simulink library "AtomicLibrary"
PostLoadFcn:
  | PacketBusGenerator; RailCabBusGenerator
(part 4 of 8)

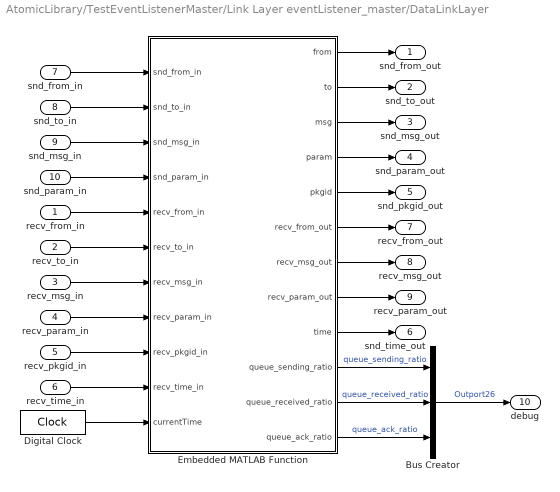
== system AtomicLibrary/TestEventListenerMaster/Link Layer eventListener_master/DataLinkLayer ==
  recv_from_in : Inport  Tag=id=_q-qdMPdmEeGH_6eRdlYQdA  Port=1  PortDimensions=-1  DataType=uint8  OutDataType=fixdt(1, 16)  OutScaling=2^0  OutDataTypeStr=uint8
  recv_to_in : Inport  Tag=id=_q-rrUPdmEeGH_6eRdlYQdA  Port=2  PortDimensions=-1  DataType=uint8  OutDataType=fixdt(1, 16)  OutScaling=2^0  OutDataTypeStr=uint8
  recv_msg_in : Inport  Tag=id=_q-sSYPdmEeGH_6eRdlYQdA  Port=3  PortDimensions=-1  DataType=uint16  OutDataType=fixdt(1, 16)  OutScaling=2^0  OutDataTypeStr=uint16
  recv_param_in : Inport  Tag=id=_q-tggPdmEeGH_6eRdlYQdA  Port=4  PortDimensions=-1  DataType=double  OutDataType=fixdt(1, 16)  OutScaling=2^0  OutDataTypeStr=double
  recv_pkgid_in : Inport  Tag=id=_q-uuoPdmEeGH_6eRdlYQdA  Port=5  PortDimensions=-1  DataType=uint32  OutDataType=fixdt(1, 16)  OutScaling=2^0  OutDataTypeStr=uint32
  recv_time_in : Inport  Tag=id=_q-v8wPdmEeGH_6eRdlYQdA  Port=6  PortDimensions=-1  DataType=double  OutDataType=fixdt(1, 16)  OutScaling=2^0  OutDataTypeStr=double
  snd_from_in : Inport  Tag=id=_q-wj0PdmEeGH_6eRdlYQdA  Port=7  PortDimensions=-1  DataType=uint8  OutDataType=fixdt(1, 16)  OutScaling=2^0  OutDataTypeStr=uint8
  snd_to_in : Inport  Tag=id=_q-xx8PdmEeGH_6eRdlYQdA  Port=8  PortDimensions=-1  DataType=uint8  OutDataType=fixdt(1, 16)  OutScaling=2^0  OutDataTypeStr=uint8
  snd_msg_in : Inport  Tag=id=_q-zAEPdmEeGH_6eRdlYQdA  Port=9  PortDimensions=-1  DataType=uint16  OutDataType=fixdt(1, 16)  OutScaling=2^0  OutDataTypeStr=uint16
  snd_param_in : Inport  Tag=id=_q-01QPdmEeGH_6eRdlYQdA  Port=10  PortDimensions=-1  DataType=double  OutDataType=fixdt(1, 16)  OutScaling=2^0  OutDataTypeStr=double
  snd_from_out : Outport  Tag=id=_q-gFIPdmEeGH_6eRdlYQdA  Port=1  PortDimensions=-1  DataType=uint8  OutDataType=fixdt(1, 16)  OutScaling=2^0  OutDataTypeStr=uint8
  snd_to_out : Outport  Tag=id=_q-gsMPdmEeGH_6eRdlYQdA  Port=2  PortDimensions=-1  DataType=uint8  OutDataType=fixdt(1, 16)  OutScaling=2^0  OutDataTypeStr=uint8
  snd_msg_out : Outport  Tag=id=_q-hTQPdmEeGH_6eRdlYQdA  Port=3  PortDimensions=-1  DataType=uint16  OutDataType=fixdt(1, 16)  OutScaling=2^0  OutDataTypeStr=uint16
  snd_param_out : Outport  Tag=id=_q-ihYPdmEeGH_6eRdlYQdA  Port=4  PortDimensions=-1  DataType=double  OutDataType=fixdt(1, 16)  OutScaling=2^0  OutDataTypeStr=double
  snd_pkgid_out : Outport  Tag=id=_q-jvgPdmEeGH_6eRdlYQdA  Port=5  PortDimensions=-1  DataType=uint32  OutDataType=fixdt(1, 16)  OutScaling=2^0  OutDataTypeStr=uint32
  snd_time_out : Outport  Tag=id=_q-k9oPdmEeGH_6eRdlYQdA  Port=6  PortDimensions=-1  DataType=double  OutDataType=fixdt(1, 16)  OutScaling=2^0  OutDataTypeStr=double
  recv_from_out : Outport  Tag=id=_q-mLwPdmEeGH_6eRdlYQdA  Port=7  PortDimensions=-1  DataType=uint8  OutDataType=fixdt(1, 16)  OutScaling=2^0  OutDataTypeStr=uint8
  recv_msg_out : Outport  Tag=id=_q-nZ4PdmEeGH_6eRdlYQdA  Port=8  PortDimensions=-1  DataType=uint16  OutDataType=fixdt(1, 16)  OutScaling=2^0  OutDataTypeStr=uint16
  recv_param_out : Outport  Tag=id=_q-oA8PdmEeGH_6eRdlYQdA  Port=9  PortDimensions=-1  DataType=double  OutDataType=fixdt(1, 16)  OutScaling=2^0  OutDataTypeStr=double
  debug : Outport  Tag=id=_q-pPEPdmEeGH_6eRdlYQdA  Port=10  PortDimensions=-1  DataType=auto  OutDataType=fixdt(1, 16)  OutScaling=2^0  OutDataTypeStr=Inherit: auto
  Bus Creator : BusCreator  Inputs=3  Tag=id=_q-2DYPdmEeGH_6eRdlYQdA
  Embedded MATLAB Function : Stateflow chart  Tag=id=_q-2DYfdmEeGH_6eRdlYQdA
  Digital Clock : DigitalClock  Tag=id=_q-5GsPdmEeGH_6eRdlYQdA  SampleTime=0.1
  wires:
  Embedded MATLAB Function/12(queue_ack_ratio) -> Bus Creator/3  "queue_ack_ratio"
  Embedded MATLAB Function/10(queue_sending_ratio) -> Bus Creator/1  "queue_sending_ratio"
  Embedded MATLAB Function/8(recv_param_out) -> recv_param_out/1
  recv_to_in/1 -> Embedded MATLAB Function/6(recv_to_in)
  Embedded MATLAB Function/5(pkgid) -> snd_pkgid_out/1
  snd_from_in/1 -> Embedded MATLAB Function/1(snd_from_in)
  Embedded MATLAB Function/7(recv_msg_out) -> recv_msg_out/1
  recv_pkgid_in/1 -> Embedded MATLAB Function/9(recv_pkgid_in)
  snd_msg_in/1 -> Embedded MATLAB Function/3(snd_msg_in)
  Digital Clock/1 -> Embedded MATLAB Function/11(currentTime)
  Embedded MATLAB Function/3(msg) -> snd_msg_out/1
  Embedded MATLAB Function/9(time) -> snd_time_out/1
  recv_from_in/1 -> Embedded MATLAB Function/5(recv_from_in)
  recv_time_in/1 -> Embedded MATLAB Function/10(recv_time_in)
  snd_to_in/1 -> Embedded MATLAB Function/2(snd_to_in)
  snd_param_in/1 -> Embedded MATLAB Function/4(snd_param_in)
  Embedded MATLAB Function/6(recv_from_out) -> recv_from_out/1
  recv_param_in/1 -> Embedded MATLAB Function/8(recv_param_in)
  Embedded MATLAB Function/2(to) -> snd_to_out/1
  recv_msg_in/1 -> Embedded MATLAB Function/7(recv_msg_in)
  Embedded MATLAB Function/4(param) -> snd_param_out/1
  Embedded MATLAB Function/1(from) -> snd_from_out/1
  Bus Creator/1 -> debug/1  "Outport26"
  Embedded MATLAB Function/11(queue_received_ratio) -> Bus Creator/2  "queue_received_ratio"

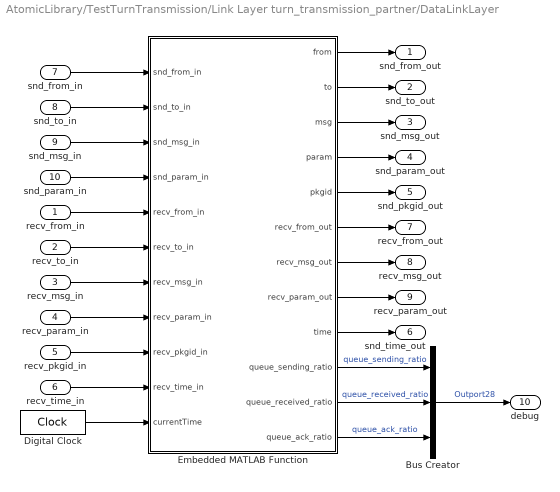
== system AtomicLibrary/TestTurnTransmission/Link Layer turn_transmission_partner/DataLinkLayer ==
  recv_from_in : Inport  Tag=id=_rHclwPdmEeGH_6eRdlYQdA  Port=1  PortDimensions=-1  DataType=uint8  OutDataType=fixdt(1, 16)  OutScaling=2^0  OutDataTypeStr=uint8
  recv_to_in : Inport  Tag=id=_rHdz4PdmEeGH_6eRdlYQdA  Port=2  PortDimensions=-1  DataType=uint8  OutDataType=fixdt(1, 16)  OutScaling=2^0  OutDataTypeStr=uint8
  recv_msg_in : Inport  Tag=id=_rHfCAPdmEeGH_6eRdlYQdA  Port=3  PortDimensions=-1  DataType=uint16  OutDataType=fixdt(1, 16)  OutScaling=2^0  OutDataTypeStr=uint16
  recv_param_in : Inport  Tag=id=_rHfpEPdmEeGH_6eRdlYQdA  Port=4  PortDimensions=-1  DataType=double  OutDataType=fixdt(1, 16)  OutScaling=2^0  OutDataTypeStr=double
  recv_pkgid_in : Inport  Tag=id=_rHg3MPdmEeGH_6eRdlYQdA  Port=5  PortDimensions=-1  DataType=uint32  OutDataType=fixdt(1, 16)  OutScaling=2^0  OutDataTypeStr=uint32
  recv_time_in : Inport  Tag=id=_rHiFUPdmEeGH_6eRdlYQdA  Port=6  PortDimensions=-1  DataType=double  OutDataType=fixdt(1, 16)  OutScaling=2^0  OutDataTypeStr=double
  snd_from_in : Inport  Tag=id=_rHjTcPdmEeGH_6eRdlYQdA  Port=7  PortDimensions=-1  DataType=uint8  OutDataType=fixdt(1, 16)  OutScaling=2^0  OutDataTypeStr=uint8
  snd_to_in : Inport  Tag=id=_rHkhkPdmEeGH_6eRdlYQdA  Port=8  PortDimensions=-1  DataType=uint8  OutDataType=fixdt(1, 16)  OutScaling=2^0  OutDataTypeStr=uint8
  snd_msg_in : Inport  Tag=id=_rHlIoPdmEeGH_6eRdlYQdA  Port=9  PortDimensions=-1  DataType=uint16  OutDataType=fixdt(1, 16)  OutScaling=2^0  OutDataTypeStr=uint16
  snd_param_in : Inport  Tag=id=_rHmWwPdmEeGH_6eRdlYQdA  Port=10  PortDimensions=-1  DataType=double  OutDataType=fixdt(1, 16)  OutScaling=2^0  OutDataTypeStr=double
  snd_from_out : Outport  Tag=id=_rHRmoPdmEeGH_6eRdlYQdA  Port=1  PortDimensions=-1  DataType=uint8  OutDataType=fixdt(1, 16)  OutScaling=2^0  OutDataTypeStr=uint8
  snd_to_out : Outport  Tag=id=_rHS0wPdmEeGH_6eRdlYQdA  Port=2  PortDimensions=-1  DataType=uint8  OutDataType=fixdt(1, 16)  OutScaling=2^0  OutDataTypeStr=uint8
  snd_msg_out : Outport  Tag=id=_rHTb0PdmEeGH_6eRdlYQdA  Port=3  PortDimensions=-1  DataType=uint16  OutDataType=fixdt(1, 16)  OutScaling=2^0  OutDataTypeStr=uint16
  snd_param_out : Outport  Tag=id=_rHUp8PdmEeGH_6eRdlYQdA  Port=4  PortDimensions=-1  DataType=double  OutDataType=fixdt(1, 16)  OutScaling=2^0  OutDataTypeStr=double
  snd_pkgid_out : Outport  Tag=id=_rHVRAPdmEeGH_6eRdlYQdA  Port=5  PortDimensions=-1  DataType=uint32  OutDataType=fixdt(1, 16)  OutScaling=2^0  OutDataTypeStr=uint32
  snd_time_out : Outport  Tag=id=_rHWfIPdmEeGH_6eRdlYQdA  Port=6  PortDimensions=-1  DataType=double  OutDataType=fixdt(1, 16)  OutScaling=2^0  OutDataTypeStr=double
  recv_from_out : Outport  Tag=id=_rHXGMPdmEeGH_6eRdlYQdA  Port=7  PortDimensions=-1  DataType=uint8  OutDataType=fixdt(1, 16)  OutScaling=2^0  OutDataTypeStr=uint8
  recv_msg_out : Outport  Tag=id=_rHYUUPdmEeGH_6eRdlYQdA  Port=8  PortDimensions=-1  DataType=uint16  OutDataType=fixdt(1, 16)  OutScaling=2^0  OutDataTypeStr=uint16
  recv_param_out : Outport  Tag=id=_rHZicPdmEeGH_6eRdlYQdA  Port=9  PortDimensions=-1  DataType=double  OutDataType=fixdt(1, 16)  OutScaling=2^0  OutDataTypeStr=double
  debug : Outport  Tag=id=_rHawkPdmEeGH_6eRdlYQdA  Port=10  PortDimensions=-1  DataType=auto  OutDataType=fixdt(1, 16)  OutScaling=2^0  OutDataTypeStr=Inherit: auto
  Bus Creator : BusCreator  Inputs=3  Tag=id=_rHoL8PdmEeGH_6eRdlYQdA
  Embedded MATLAB Function : Stateflow chart  Tag=id=_rHoL8fdmEeGH_6eRdlYQdA
  Digital Clock : DigitalClock  Tag=id=_rHqoMPdmEeGH_6eRdlYQdA  SampleTime=0.1
  wires:
  Embedded MATLAB Function/12(queue_ack_ratio) -> Bus Creator/3  "queue_ack_ratio"
  Embedded MATLAB Function/10(queue_sending_ratio) -> Bus Creator/1  "queue_sending_ratio"
  Embedded MATLAB Function/8(recv_param_out) -> recv_param_out/1
  recv_to_in/1 -> Embedded MATLAB Function/6(recv_to_in)
  Embedded MATLAB Function/5(pkgid) -> snd_pkgid_out/1
  snd_from_in/1 -> Embedded MATLAB Function/1(snd_from_in)
  Embedded MATLAB Function/7(recv_msg_out) -> recv_msg_out/1
  recv_pkgid_in/1 -> Embedded MATLAB Function/9(recv_pkgid_in)
  snd_msg_in/1 -> Embedded MATLAB Function/3(snd_msg_in)
  Digital Clock/1 -> Embedded MATLAB Function/11(currentTime)
  Embedded MATLAB Function/3(msg) -> snd_msg_out/1
  Embedded MATLAB Function/9(time) -> snd_time_out/1
  recv_from_in/1 -> Embedded MATLAB Function/5(recv_from_in)
  recv_time_in/1 -> Embedded MATLAB Function/10(recv_time_in)
  snd_to_in/1 -> Embedded MATLAB Function/2(snd_to_in)
  snd_param_in/1 -> Embedded MATLAB Function/4(snd_param_in)
  Embedded MATLAB Function/6(recv_from_out) -> recv_from_out/1
  recv_param_in/1 -> Embedded MATLAB Function/8(recv_param_in)
  Embedded MATLAB Function/2(to) -> snd_to_out/1
  recv_msg_in/1 -> Embedded MATLAB Function/7(recv_msg_in)
  Embedded MATLAB Function/4(param) -> snd_param_out/1
  Embedded MATLAB Function/1(from) -> snd_from_out/1
  Bus Creator/1 -> debug/1  "Outport28"
  Embedded MATLAB Function/11(queue_received_ratio) -> Bus Creator/2  "queue_received_ratio"

== system AtomicLibrary/TestRequestInformationProvider/Link Layer requestinformation_provider/DataLinkLayer ==
  recv_from_in : Inport  Tag=id=_rQl6sPdmEeGH_6eRdlYQdA  Port=1  PortDimensions=-1  DataType=uint8  OutDataType=fixdt(1, 16)  OutScaling=2^0  OutDataTypeStr=uint8
  recv_to_in : Inport  Tag=id=_rQnI0PdmEeGH_6eRdlYQdA  Port=2  PortDimensions=-1  DataType=uint8  OutDataType=fixdt(1, 16)  OutScaling=2^0  OutDataTypeStr=uint8
  recv_msg_in : Inport  Tag=id=_rQnv4PdmEeGH_6eRdlYQdA  Port=3  PortDimensions=-1  DataType=uint16  OutDataType=fixdt(1, 16)  OutScaling=2^0  OutDataTypeStr=uint16
  recv_param_in : Inport  Tag=id=_rQo-APdmEeGH_6eRdlYQdA  Port=4  PortDimensions=-1  DataType=double  OutDataType=fixdt(1, 16)  OutScaling=2^0  OutDataTypeStr=double
  recv_pkgid_in : Inport  Tag=id=_rQqMIPdmEeGH_6eRdlYQdA  Port=5  PortDimensions=-1  DataType=uint32  OutDataType=fixdt(1, 16)  OutScaling=2^0  OutDataTypeStr=uint32
  recv_time_in : Inport  Tag=id=_rQqzMPdmEeGH_6eRdlYQdA  Port=6  PortDimensions=-1  DataType=double  OutDataType=fixdt(1, 16)  OutScaling=2^0  OutDataTypeStr=double
  snd_from_in : Inport  Tag=id=_rQsBUPdmEeGH_6eRdlYQdA  Port=7  PortDimensions=-1  DataType=uint8  OutDataType=fixdt(1, 16)  OutScaling=2^0  OutDataTypeStr=uint8
  snd_to_in : Inport  Tag=id=_rQtPcPdmEeGH_6eRdlYQdA  Port=8  PortDimensions=-1  DataType=uint8  OutDataType=fixdt(1, 16)  OutScaling=2^0  OutDataTypeStr=uint8
  snd_msg_in : Inport  Tag=id=_rQudkPdmEeGH_6eRdlYQdA  Port=9  PortDimensions=-1  DataType=uint16  OutDataType=fixdt(1, 16)  OutScaling=2^0  OutDataTypeStr=uint16
  snd_param_in : Inport  Tag=id=_rQvrsPdmEeGH_6eRdlYQdA  Port=10  PortDimensions=-1  DataType=double  OutDataType=fixdt(1, 16)  OutScaling=2^0  OutDataTypeStr=double
  snd_from_out : Outport  Tag=id=_rQcwwPdmEeGH_6eRdlYQdA  Port=1  PortDimensions=-1  DataType=uint8  OutDataType=fixdt(1, 16)  OutScaling=2^0  OutDataTypeStr=uint8
  snd_to_out : Outport  Tag=id=_rQdX0PdmEeGH_6eRdlYQdA  Port=2  PortDimensions=-1  DataType=uint8  OutDataType=fixdt(1, 16)  OutScaling=2^0  OutDataTypeStr=uint8
  snd_msg_out : Outport  Tag=id=_rQel8PdmEeGH_6eRdlYQdA  Port=3  PortDimensions=-1  DataType=uint16  OutDataType=fixdt(1, 16)  OutScaling=2^0  OutDataTypeStr=uint16
  snd_param_out : Outport  Tag=id=_rQfNAPdmEeGH_6eRdlYQdA  Port=4  PortDimensions=-1  DataType=double  OutDataType=fixdt(1, 16)  OutScaling=2^0  OutDataTypeStr=double
  snd_pkgid_out : Outport  Tag=id=_rQgbIPdmEeGH_6eRdlYQdA  Port=5  PortDimensions=-1  DataType=uint32  OutDataType=fixdt(1, 16)  OutScaling=2^0  OutDataTypeStr=uint32
  snd_time_out : Outport  Tag=id=_rQhCMPdmEeGH_6eRdlYQdA  Port=6  PortDimensions=-1  DataType=double  OutDataType=fixdt(1, 16)  OutScaling=2^0  OutDataTypeStr=double
  recv_from_out : Outport  Tag=id=_rQiQUPdmEeGH_6eRdlYQdA  Port=7  PortDimensions=-1  DataType=uint8  OutDataType=fixdt(1, 16)  OutScaling=2^0  OutDataTypeStr=uint8
  recv_msg_out : Outport  Tag=id=_rQi3YPdmEeGH_6eRdlYQdA  Port=8  PortDimensions=-1  DataType=uint16  OutDataType=fixdt(1, 16)  OutScaling=2^0  OutDataTypeStr=uint16
  recv_param_out : Outport  Tag=id=_rQkFgPdmEeGH_6eRdlYQdA  Port=9  PortDimensions=-1  DataType=double  OutDataType=fixdt(1, 16)  OutScaling=2^0  OutDataTypeStr=double
  debug : Outport  Tag=id=_rQkskPdmEeGH_6eRdlYQdA  Port=10  PortDimensions=-1  DataType=auto  OutDataType=fixdt(1, 16)  OutScaling=2^0  OutDataTypeStr=Inherit: auto
  Bus Creator : BusCreator  Inputs=3  Tag=id=_rQwSwPdmEeGH_6eRdlYQdA
  Embedded MATLAB Function : Stateflow chart  Tag=id=_rQw50PdmEeGH_6eRdlYQdA
  Digital Clock : DigitalClock  Tag=id=_rQzWEPdmEeGH_6eRdlYQdA  SampleTime=0.1
  wires:
  Embedded MATLAB Function/12(queue_ack_ratio) -> Bus Creator/3  "queue_ack_ratio"
  Embedded MATLAB Function/10(queue_sending_ratio) -> Bus Creator/1  "queue_sending_ratio"
  Embedded MATLAB Function/8(recv_param_out) -> recv_param_out/1
  recv_to_in/1 -> Embedded MATLAB Function/6(recv_to_in)
  Embedded MATLAB Function/5(pkgid) -> snd_pkgid_out/1
  snd_from_in/1 -> Embedded MATLAB Function/1(snd_from_in)
  Embedded MATLAB Function/7(recv_msg_out) -> recv_msg_out/1
  recv_pkgid_in/1 -> Embedded MATLAB Function/9(recv_pkgid_in)
  snd_msg_in/1 -> Embedded MATLAB Function/3(snd_msg_in)
  Digital Clock/1 -> Embedded MATLAB Function/11(currentTime)
  Embedded MATLAB Function/3(msg) -> snd_msg_out/1
  Embedded MATLAB Function/9(time) -> snd_time_out/1
  recv_from_in/1 -> Embedded MATLAB Function/5(recv_from_in)
  recv_time_in/1 -> Embedded MATLAB Function/10(recv_time_in)
  snd_to_in/1 -> Embedded MATLAB Function/2(snd_to_in)
  snd_param_in/1 -> Embedded MATLAB Function/4(snd_param_in)
  Embedded MATLAB Function/6(recv_from_out) -> recv_from_out/1
  recv_param_in/1 -> Embedded MATLAB Function/8(recv_param_in)
  Embedded MATLAB Function/2(to) -> snd_to_out/1
  recv_msg_in/1 -> Embedded MATLAB Function/7(recv_msg_in)
  Embedded MATLAB Function/4(param) -> snd_param_out/1
  Embedded MATLAB Function/1(from) -> snd_from_out/1
  Bus Creator/1 -> debug/1  "Outport30"
  Embedded MATLAB Function/11(queue_received_ratio) -> Bus Creator/2  "queue_received_ratio"

== system AtomicLibrary/TestRequestInformaitonUser/Link Layer requestinformation_user/DataLinkLayer ==
  recv_from_in : Inport  Tag=id=_rZHkkPdmEeGH_6eRdlYQdA  Port=1  PortDimensions=-1  DataType=uint8  OutDataType=fixdt(1, 16)  OutScaling=2^0  OutDataTypeStr=uint8
  recv_to_in : Inport  Tag=id=_rZILoPdmEeGH_6eRdlYQdA  Port=2  PortDimensions=-1  DataType=uint8  OutDataType=fixdt(1, 16)  OutScaling=2^0  OutDataTypeStr=uint8
  recv_msg_in : Inport  Tag=id=_rZKA0PdmEeGH_6eRdlYQdA  Port=3  PortDimensions=-1  DataType=uint16  OutDataType=fixdt(1, 16)  OutScaling=2^0  OutDataTypeStr=uint16
  recv_param_in : Inport  Tag=id=_rZLO8PdmEeGH_6eRdlYQdA  Port=4  PortDimensions=-1  DataType=double  OutDataType=fixdt(1, 16)  OutScaling=2^0  OutDataTypeStr=double
  recv_pkgid_in : Inport  Tag=id=_rZMdEPdmEeGH_6eRdlYQdA  Port=5  PortDimensions=-1  DataType=uint32  OutDataType=fixdt(1, 16)  OutScaling=2^0  OutDataTypeStr=uint32
  recv_time_in : Inport  Tag=id=_rZNrMPdmEeGH_6eRdlYQdA  Port=6  PortDimensions=-1  DataType=double  OutDataType=fixdt(1, 16)  OutScaling=2^0  OutDataTypeStr=double
  snd_from_in : Inport  Tag=id=_rZOSQPdmEeGH_6eRdlYQdA  Port=7  PortDimensions=-1  DataType=uint8  OutDataType=fixdt(1, 16)  OutScaling=2^0  OutDataTypeStr=uint8
  snd_to_in : Inport  Tag=id=_rZPgYPdmEeGH_6eRdlYQdA  Port=8  PortDimensions=-1  DataType=uint8  OutDataType=fixdt(1, 16)  OutScaling=2^0  OutDataTypeStr=uint8
  snd_msg_in : Inport  Tag=id=_rZRVkPdmEeGH_6eRdlYQdA  Port=9  PortDimensions=-1  DataType=uint16  OutDataType=fixdt(1, 16)  OutScaling=2^0  OutDataTypeStr=uint16
  snd_param_in : Inport  Tag=id=_rZSjsPdmEeGH_6eRdlYQdA  Port=10  PortDimensions=-1  DataType=double  OutDataType=fixdt(1, 16)  OutScaling=2^0  OutDataTypeStr=double
  snd_from_out : Outport  Tag=id=_rY9zkPdmEeGH_6eRdlYQdA  Port=1  PortDimensions=-1  DataType=uint8  OutDataType=fixdt(1, 16)  OutScaling=2^0  OutDataTypeStr=uint8
  snd_to_out : Outport  Tag=id=_rY-aoPdmEeGH_6eRdlYQdA  Port=2  PortDimensions=-1  DataType=uint8  OutDataType=fixdt(1, 16)  OutScaling=2^0  OutDataTypeStr=uint8
  snd_msg_out : Outport  Tag=id=_rY_owPdmEeGH_6eRdlYQdA  Port=3  PortDimensions=-1  DataType=uint16  OutDataType=fixdt(1, 16)  OutScaling=2^0  OutDataTypeStr=uint16
  snd_param_out : Outport  Tag=id=_rZAP0PdmEeGH_6eRdlYQdA  Port=4  PortDimensions=-1  DataType=double  OutDataType=fixdt(1, 16)  OutScaling=2^0  OutDataTypeStr=double
  snd_pkgid_out : Outport  Tag=id=_rZBd8PdmEeGH_6eRdlYQdA  Port=5  PortDimensions=-1  DataType=uint32  OutDataType=fixdt(1, 16)  OutScaling=2^0  OutDataTypeStr=uint32
  snd_time_out : Outport  Tag=id=_rZCFAPdmEeGH_6eRdlYQdA  Port=6  PortDimensions=-1  DataType=double  OutDataType=fixdt(1, 16)  OutScaling=2^0  OutDataTypeStr=double
  recv_from_out : Outport  Tag=id=_rZDTIPdmEeGH_6eRdlYQdA  Port=7  PortDimensions=-1  DataType=uint8  OutDataType=fixdt(1, 16)  OutScaling=2^0  OutDataTypeStr=uint8
  recv_msg_out : Outport  Tag=id=_rZEhQPdmEeGH_6eRdlYQdA  Port=8  PortDimensions=-1  DataType=uint16  OutDataType=fixdt(1, 16)  OutScaling=2^0  OutDataTypeStr=uint16
  recv_param_out : Outport  Tag=id=_rZFIUPdmEeGH_6eRdlYQdA  Port=9  PortDimensions=-1  DataType=double  OutDataType=fixdt(1, 16)  OutScaling=2^0  OutDataTypeStr=double
  debug : Outport  Tag=id=_rZGWcPdmEeGH_6eRdlYQdA  Port=10  PortDimensions=-1  DataType=auto  OutDataType=fixdt(1, 16)  OutScaling=2^0  OutDataTypeStr=Inherit: auto
  Bus Creator : BusCreator  Inputs=3  Tag=id=_rZTx0PdmEeGH_6eRdlYQdA
  Embedded MATLAB Function : Stateflow chart  Tag=id=_rZTx0fdmEeGH_6eRdlYQdA
  Digital Clock : DigitalClock  Tag=id=_rZWOEPdmEeGH_6eRdlYQdA  SampleTime=0.1
  wires:
  Embedded MATLAB Function/12(queue_ack_ratio) -> Bus Creator/3  "queue_ack_ratio"
  Embedded MATLAB Function/10(queue_sending_ratio) -> Bus Creator/1  "queue_sending_ratio"
  Embedded MATLAB Function/8(recv_param_out) -> recv_param_out/1
  recv_to_in/1 -> Embedded MATLAB Function/6(recv_to_in)
  Embedded MATLAB Function/5(pkgid) -> snd_pkgid_out/1
  snd_from_in/1 -> Embedded MATLAB Function/1(snd_from_in)
  Embedded MATLAB Function/7(recv_msg_out) -> recv_msg_out/1
  recv_pkgid_in/1 -> Embedded MATLAB Function/9(recv_pkgid_in)
  snd_msg_in/1 -> Embedded MATLAB Function/3(snd_msg_in)
  Digital Clock/1 -> Embedded MATLAB Function/11(currentTime)
  Embedded MATLAB Function/3(msg) -> snd_msg_out/1
  Embedded MATLAB Function/9(time) -> snd_time_out/1
  recv_from_in/1 -> Embedded MATLAB Function/5(recv_from_in)
  recv_time_in/1 -> Embedded MATLAB Function/10(recv_time_in)
  snd_to_in/1 -> Embedded MATLAB Function/2(snd_to_in)
  snd_param_in/1 -> Embedded MATLAB Function/4(snd_param_in)
  Embedded MATLAB Function/6(recv_from_out) -> recv_from_out/1
  recv_param_in/1 -> Embedded MATLAB Function/8(recv_param_in)
  Embedded MATLAB Function/2(to) -> snd_to_out/1
  recv_msg_in/1 -> Embedded MATLAB Function/7(recv_msg_in)
  Embedded MATLAB Function/4(param) -> snd_param_out/1
  Embedded MATLAB Function/1(from) -> snd_from_out/1
  Bus Creator/1 -> debug/1  "Outport32"
  Embedded MATLAB Function/11(queue_received_ratio) -> Bus Creator/2  "queue_received_ratio"

== system AtomicLibrary/TestStartStopSlave/Link Layer startStop_Slave/DataLinkLayer ==
  recv_from_in : Inport  Tag=id=_riEFMPdmEeGH_6eRdlYQdA  Port=1  PortDimensions=-1  DataType=uint8  OutDataType=fixdt(1, 16)  OutScaling=2^0  OutDataTypeStr=uint8
  recv_to_in : Inport  Tag=id=_riFTUPdmEeGH_6eRdlYQdA  Port=2  PortDimensions=-1  DataType=uint8  OutDataType=fixdt(1, 16)  OutScaling=2^0  OutDataTypeStr=uint8
  recv_msg_in : Inport  Tag=id=_riGhcPdmEeGH_6eRdlYQdA  Port=3  PortDimensions=-1  DataType=uint16  OutDataType=fixdt(1, 16)  OutScaling=2^0  OutDataTypeStr=uint16
  recv_param_in : Inport  Tag=id=_riHvkPdmEeGH_6eRdlYQdA  Port=4  PortDimensions=-1  DataType=double  OutDataType=fixdt(1, 16)  OutScaling=2^0  OutDataTypeStr=double
  recv_pkgid_in : Inport  Tag=id=_riI9sPdmEeGH_6eRdlYQdA  Port=5  PortDimensions=-1  DataType=uint32  OutDataType=fixdt(1, 16)  OutScaling=2^0  OutDataTypeStr=uint32
  recv_time_in : Inport  Tag=id=_riKL0PdmEeGH_6eRdlYQdA  Port=6  PortDimensions=-1  DataType=double  OutDataType=fixdt(1, 16)  OutScaling=2^0  OutDataTypeStr=double
  snd_from_in : Inport  Tag=id=_riKy4PdmEeGH_6eRdlYQdA  Port=7  PortDimensions=-1  DataType=uint8  OutDataType=fixdt(1, 16)  OutScaling=2^0  OutDataTypeStr=uint8
  snd_to_in : Inport  Tag=id=_riMBAPdmEeGH_6eRdlYQdA  Port=8  PortDimensions=-1  DataType=uint8  OutDataType=fixdt(1, 16)  OutScaling=2^0  OutDataTypeStr=uint8
  snd_msg_in : Inport  Tag=id=_riN2MPdmEeGH_6eRdlYQdA  Port=9  PortDimensions=-1  DataType=uint16  OutDataType=fixdt(1, 16)  OutScaling=2^0  OutDataTypeStr=uint16
  snd_param_in : Inport  Tag=id=_riPrYPdmEeGH_6eRdlYQdA  Port=10  PortDimensions=-1  DataType=double  OutDataType=fixdt(1, 16)  OutScaling=2^0  OutDataTypeStr=double
  snd_from_out : Outport  Tag=id=_rh5tIPdmEeGH_6eRdlYQdA  Port=1  PortDimensions=-1  DataType=uint8  OutDataType=fixdt(1, 16)  OutScaling=2^0  OutDataTypeStr=uint8
  snd_to_out : Outport  Tag=id=_rh67QPdmEeGH_6eRdlYQdA  Port=2  PortDimensions=-1  DataType=uint8  OutDataType=fixdt(1, 16)  OutScaling=2^0  OutDataTypeStr=uint8
  snd_msg_out : Outport  Tag=id=_rh8JYPdmEeGH_6eRdlYQdA  Port=3  PortDimensions=-1  DataType=uint16  OutDataType=fixdt(1, 16)  OutScaling=2^0  OutDataTypeStr=uint16
  snd_param_out : Outport  Tag=id=_rh8wcPdmEeGH_6eRdlYQdA  Port=4  PortDimensions=-1  DataType=double  OutDataType=fixdt(1, 16)  OutScaling=2^0  OutDataTypeStr=double
  snd_pkgid_out : Outport  Tag=id=_rh9-kPdmEeGH_6eRdlYQdA  Port=5  PortDimensions=-1  DataType=uint32  OutDataType=fixdt(1, 16)  OutScaling=2^0  OutDataTypeStr=uint32
  snd_time_out : Outport  Tag=id=_rh-loPdmEeGH_6eRdlYQdA  Port=6  PortDimensions=-1  DataType=double  OutDataType=fixdt(1, 16)  OutScaling=2^0  OutDataTypeStr=double
  recv_from_out : Outport  Tag=id=_rh_zwPdmEeGH_6eRdlYQdA  Port=7  PortDimensions=-1  DataType=uint8  OutDataType=fixdt(1, 16)  OutScaling=2^0  OutDataTypeStr=uint8
  recv_msg_out : Outport  Tag=id=_riBB4PdmEeGH_6eRdlYQdA  Port=8  PortDimensions=-1  DataType=uint16  OutDataType=fixdt(1, 16)  OutScaling=2^0  OutDataTypeStr=uint16
  recv_param_out : Outport  Tag=id=_riCQAPdmEeGH_6eRdlYQdA  Port=9  PortDimensions=-1  DataType=double  OutDataType=fixdt(1, 16)  OutScaling=2^0  OutDataTypeStr=double
  debug : Outport  Tag=id=_riC3EPdmEeGH_6eRdlYQdA  Port=10  PortDimensions=-1  DataType=auto  OutDataType=fixdt(1, 16)  OutScaling=2^0  OutDataTypeStr=Inherit: auto
  Bus Creator : BusCreator  Inputs=3  Tag=id=_riRgkPdmEeGH_6eRdlYQdA
  Embedded MATLAB Function : Stateflow chart  Tag=id=_riRgkfdmEeGH_6eRdlYQdA
  Digital Clock : DigitalClock  Tag=id=_riT80PdmEeGH_6eRdlYQdA  SampleTime=0.1
  wires:
  Embedded MATLAB Function/12(queue_ack_ratio) -> Bus Creator/3  "queue_ack_ratio"
  Embedded MATLAB Function/10(queue_sending_ratio) -> Bus Creator/1  "queue_sending_ratio"
  Embedded MATLAB Function/8(recv_param_out) -> recv_param_out/1
  recv_to_in/1 -> Embedded MATLAB Function/6(recv_to_in)
  Embedded MATLAB Function/5(pkgid) -> snd_pkgid_out/1
  snd_from_in/1 -> Embedded MATLAB Function/1(snd_from_in)
  Embedded MATLAB Function/7(recv_msg_out) -> recv_msg_out/1
  recv_pkgid_in/1 -> Embedded MATLAB Function/9(recv_pkgid_in)
  snd_msg_in/1 -> Embedded MATLAB Function/3(snd_msg_in)
  Digital Clock/1 -> Embedded MATLAB Function/11(currentTime)
  Embedded MATLAB Function/3(msg) -> snd_msg_out/1
  Embedded MATLAB Function/9(time) -> snd_time_out/1
  recv_from_in/1 -> Embedded MATLAB Function/5(recv_from_in)
  recv_time_in/1 -> Embedded MATLAB Function/10(recv_time_in)
  snd_to_in/1 -> Embedded MATLAB Function/2(snd_to_in)
  snd_param_in/1 -> Embedded MATLAB Function/4(snd_param_in)
  Embedded MATLAB Function/6(recv_from_out) -> recv_from_out/1
  recv_param_in/1 -> Embedded MATLAB Function/8(recv_param_in)
  Embedded MATLAB Function/2(to) -> snd_to_out/1
  recv_msg_in/1 -> Embedded MATLAB Function/7(recv_msg_in)
  Embedded MATLAB Function/4(param) -> snd_param_out/1
  Embedded MATLAB Function/1(from) -> snd_from_out/1
  Bus Creator/1 -> debug/1  "Outport34"
  Embedded MATLAB Function/11(queue_received_ratio) -> Bus Creator/2  "queue_received_ratio"

== system AtomicLibrary/TestStartStopMaster/Link Layer startStop_Master/DataLinkLayer ==
  recv_from_in : Inport  Tag=id=_rrbckPdmEeGH_6eRdlYQdA  Port=1  PortDimensions=-1  DataType=uint8  OutDataType=fixdt(1, 16)  OutScaling=2^0  OutDataTypeStr=uint8
  recv_to_in : Inport  Tag=id=_rrcqsPdmEeGH_6eRdlYQdA  Port=2  PortDimensions=-1  DataType=uint8  OutDataType=fixdt(1, 16)  OutScaling=2^0  OutDataTypeStr=uint8
  recv_msg_in : Inport  Tag=id=_rrdRwPdmEeGH_6eRdlYQdA  Port=3  PortDimensions=-1  DataType=uint16  OutDataType=fixdt(1, 16)  OutScaling=2^0  OutDataTypeStr=uint16
  recv_param_in : Inport  Tag=id=_rref4PdmEeGH_6eRdlYQdA  Port=4  PortDimensions=-1  DataType=double  OutDataType=fixdt(1, 16)  OutScaling=2^0  OutDataTypeStr=double
  recv_pkgid_in : Inport  Tag=id=_rrfuAPdmEeGH_6eRdlYQdA  Port=5  PortDimensions=-1  DataType=uint32  OutDataType=fixdt(1, 16)  OutScaling=2^0  OutDataTypeStr=uint32
  recv_time_in : Inport  Tag=id=_rrg8IPdmEeGH_6eRdlYQdA  Port=6  PortDimensions=-1  DataType=double  OutDataType=fixdt(1, 16)  OutScaling=2^0  OutDataTypeStr=double
  snd_from_in : Inport  Tag=id=_rriKQPdmEeGH_6eRdlYQdA  Port=7  PortDimensions=-1  DataType=uint8  OutDataType=fixdt(1, 16)  OutScaling=2^0  OutDataTypeStr=uint8
  snd_to_in : Inport  Tag=id=_rrixUPdmEeGH_6eRdlYQdA  Port=8  PortDimensions=-1  DataType=uint8  OutDataType=fixdt(1, 16)  OutScaling=2^0  OutDataTypeStr=uint8
  snd_msg_in : Inport  Tag=id=_rrj_cPdmEeGH_6eRdlYQdA  Port=9  PortDimensions=-1  DataType=uint16  OutDataType=fixdt(1, 16)  OutScaling=2^0  OutDataTypeStr=uint16
  snd_param_in : Inport  Tag=id=_rrlNkPdmEeGH_6eRdlYQdA  Port=10  PortDimensions=-1  DataType=double  OutDataType=fixdt(1, 16)  OutScaling=2^0  OutDataTypeStr=double
  snd_from_out : Outport  Tag=id=_rrOoQPdmEeGH_6eRdlYQdA  Port=1  PortDimensions=-1  DataType=uint8  OutDataType=fixdt(1, 16)  OutScaling=2^0  OutDataTypeStr=uint8
  snd_to_out : Outport  Tag=id=_rrQdcPdmEeGH_6eRdlYQdA  Port=2  PortDimensions=-1  DataType=uint8  OutDataType=fixdt(1, 16)  OutScaling=2^0  OutDataTypeStr=uint8
  snd_msg_out : Outport  Tag=id=_rrRrkPdmEeGH_6eRdlYQdA  Port=3  PortDimensions=-1  DataType=uint16  OutDataType=fixdt(1, 16)  OutScaling=2^0  OutDataTypeStr=uint16
  snd_param_out : Outport  Tag=id=_rrTgwPdmEeGH_6eRdlYQdA  Port=4  PortDimensions=-1  DataType=double  OutDataType=fixdt(1, 16)  OutScaling=2^0  OutDataTypeStr=double
  snd_pkgid_out : Outport  Tag=id=_rrUu4PdmEeGH_6eRdlYQdA  Port=5  PortDimensions=-1  DataType=uint32  OutDataType=fixdt(1, 16)  OutScaling=2^0  OutDataTypeStr=uint32
  snd_time_out : Outport  Tag=id=_rrV9APdmEeGH_6eRdlYQdA  Port=6  PortDimensions=-1  DataType=double  OutDataType=fixdt(1, 16)  OutScaling=2^0  OutDataTypeStr=double
  recv_from_out : Outport  Tag=id=_rrXLIPdmEeGH_6eRdlYQdA  Port=7  PortDimensions=-1  DataType=uint8  OutDataType=fixdt(1, 16)  OutScaling=2^0  OutDataTypeStr=uint8
  recv_msg_out : Outport  Tag=id=_rrYZQPdmEeGH_6eRdlYQdA  Port=8  PortDimensions=-1  DataType=uint16  OutDataType=fixdt(1, 16)  OutScaling=2^0  OutDataTypeStr=uint16
  recv_param_out : Outport  Tag=id=_rrZnYPdmEeGH_6eRdlYQdA  Port=9  PortDimensions=-1  DataType=double  OutDataType=fixdt(1, 16)  OutScaling=2^0  OutDataTypeStr=double
  debug : Outport  Tag=id=_rraOcPdmEeGH_6eRdlYQdA  Port=10  PortDimensions=-1  DataType=auto  OutDataType=fixdt(1, 16)  OutScaling=2^0  OutDataTypeStr=Inherit: auto
  Bus Creator : BusCreator  Inputs=3  Tag=id=_rrmbsPdmEeGH_6eRdlYQdA
  Embedded MATLAB Function : Stateflow chart  Tag=id=_rrnCwPdmEeGH_6eRdlYQdA
  Digital Clock : DigitalClock  Tag=id=_rro38PdmEeGH_6eRdlYQdA  SampleTime=0.1
  wires:
  Embedded MATLAB Function/12(queue_ack_ratio) -> Bus Creator/3  "queue_ack_ratio"
  Embedded MATLAB Function/10(queue_sending_ratio) -> Bus Creator/1  "queue_sending_ratio"
  Embedded MATLAB Function/8(recv_param_out) -> recv_param_out/1
  recv_to_in/1 -> Embedded MATLAB Function/6(recv_to_in)
  Embedded MATLAB Function/5(pkgid) -> snd_pkgid_out/1
  snd_from_in/1 -> Embedded MATLAB Function/1(snd_from_in)
  Embedded MATLAB Function/7(recv_msg_out) -> recv_msg_out/1
  recv_pkgid_in/1 -> Embedded MATLAB Function/9(recv_pkgid_in)
  snd_msg_in/1 -> Embedded MATLAB Function/3(snd_msg_in)
  Digital Clock/1 -> Embedded MATLAB Function/11(currentTime)
  Embedded MATLAB Function/3(msg) -> snd_msg_out/1
  Embedded MATLAB Function/9(time) -> snd_time_out/1
  recv_from_in/1 -> Embedded MATLAB Function/5(recv_from_in)
  recv_time_in/1 -> Embedded MATLAB Function/10(recv_time_in)
  snd_to_in/1 -> Embedded MATLAB Function/2(snd_to_in)
  snd_param_in/1 -> Embedded MATLAB Function/4(snd_param_in)
  Embedded MATLAB Function/6(recv_from_out) -> recv_from_out/1
  recv_param_in/1 -> Embedded MATLAB Function/8(recv_param_in)
  Embedded MATLAB Function/2(to) -> snd_to_out/1
  recv_msg_in/1 -> Embedded MATLAB Function/7(recv_msg_in)
  Embedded MATLAB Function/4(param) -> snd_param_out/1
  Embedded MATLAB Function/1(from) -> snd_from_out/1
  Bus Creator/1 -> debug/1  "Outport36"
  Embedded MATLAB Function/11(queue_received_ratio) -> Bus Creator/2  "queue_received_ratio"

== stateflow chart TestDelegationSlave/TestDelegationSlave_Statechart ==
  state chart
    state chartRegion [parallel]
      state Main
        state synchronization [parallel]
          state Waiting
            entry: beginAvailableStatechart = true
            exit: beginAvailableStatechart = false
          state s1
          state s2
          Waiting -> s1 : begin
          s1 -> s2 : [successAvailablePortDelegSlave]{send(success, portDelegSlave)}
        state portDelegSlave [parallel]
          state Inactive
          state Success
          state Fail
          state Running
            entry: successAvailableDelegation_Slave = true; failureAvailableDelegation_Slave = true; reset(c0)
            exit: successAvailableDelegation_Slave = false; failureAvailableDelegation_Slave = false
          state Inv_Error
          Success -> Inactive [order 1] : {[delegation_slaveEvtWriteOut, delegation_slaveParamWriteOut] = enqueue(EVT_COMPLETED, delegation_slaveEvtWriteOut, delegation_slaveParamWriteOut)}
          Fail -> Inactive [order 1] : {[delegation_slaveEvtWriteOut, delegation_slaveParamWriteOut] = enqueue(EVT_FAILED, delegation_slaveEvtWriteOut, delegation_slaveParamWriteOut)}
          Running -> Success [order 2] : success
          Running -> Fail [order 1] : failure
          Inactive -> Running : [(beginAvailableSynchronization) && ([checkQueue(EVT_DELEGATE, delegation_slaveEvtReadOut)])]{send(begin, synchronization)}
          Success -> Inv_Error [order 2] : [time(c0) > 20]
          Fail -> Inv_Error [order 2] : [time(c0) > 20]
          Running -> Inv_Error [order 3] : [time(c0) > 20]
    state DataInit [parallel]
    DataInit -> DataInit : {delegation_slaveEvtWriteOut = delegation_slaveEvtWriteIn;
        | delegation_slaveParamWriteOut = delegation_slaveParamWriteIn;
        | delegation_slaveEvtReadOut = delegation_slaveEvtReadIn;
        | delegation_slaveParamReadOut = delegation_slaveParamReadIn;
        | }
  (default) -> Waiting
  (default) -> Inactive
  (default) -> Main
  (default) -> chart
  data: EVT_DELEGATE constant uint32 =2; EVT_COMPLETED constant uint32 =3; EVT_FAILED constant uint32 =4; c0 local double =0.0; EVT_COMPLETED constant uint32 =3; EVT_FAILED constant uint32 =4; EVT_DELEGATE constant uint32 =2; beginAvailableStatechart local boolean =false; successAvailableDelegation_Slave local boolean =false; failureAvailableDelegation_Slave local boolean =false; evtQueueIn function_input; param function_input; paramQueueIn function_input; event function_input; evtQueue function_output; paramQueue function_output; event function_input; evtQueue function_input; available function_output; event function_input; evtQueueIn function_input; paramQueueIn function_input; evtQueue function_output; paramQueue function_output; parameter function_output; clock function_input; logicalTime function_output; clock function_input; clockSignal input; delegation_slaveReadIn input; delegation_slaveParamReadIn input; delegation_slaveWriteIn input; delegation_slaveParamWriteIn input; delegation_slaveReadOut output; delegation_slaveParamReadOut output; delegation_slaveWriteOut output; delegation_slaveParamWriteOut output
  events: begin local EITHER_EDGE_EVENT; failure local EITHER_EDGE_EVENT; success local EITHER_EDGE_EVENT
  function enqueue:
    | function [evtQueue, paramQueue] = enqueue(event, evtQueueIn, param, paramQueueIn) %eml 
    |  evtQueue = evtQueueIn; 
    |  paramQueue = paramQueueIn; 
    |  for i = 1:length(evtQueueIn) 
    |  if evtQueueIn(i) == uint8(0) 
    |  evtQueueIn(i) = event; 
    |  paramQueue(i) = param; 
    |  return 
    |  end 
    |  end
  function checkQueue:
    | function available = checkQueue(event, evtQueue) %eml 
    |  available = false; 
    |  for i = 1:length(evtQueue) 
    |      if evtQueue(i) == event 
    |          available = true;    
    |          return 
    |      end 
    |  end
  function dequeue:
    | function [evtQueue, paramQueue, parameter] = dequeue(event, evtQueueIn, paramQueueIn) %eml 
    |  evtQueue = evtQueueIn; 
    |  paramQueue = paramQueueIn; 
    |  parameter = 0; 
    |  for i = 1:length(evtQueue) 
    |  if evtQueue(i) == event 
    |  parameter = paramQueue(i); 
    |  for j = i:length(evtQueue)-1 
    |   evtQueue(j) = evtQueue(j+1); 
    |  paramQueue(j) = paramQueue(j+1); 
    |  end 
    |  evtQueue(length(evtQueue)) = 0; 
    |  paramQueue(length(paramQueue)) = 0; 
    |  return 
    |  end 
    |  end
  function time:
    | function logicalTime = time(clock) 
    |  sample = 0.01;  % the sample time of the system clock 
    |  %convert to pass units of time after last reset 
    |  logicalTime = uint32((clockSignal - clock)/sample);
  function reset:
    | function reset(clock) 
    |  %set clock variable to current time 
    |  clock = clockSignal;

== stateflow chart TestDelegationMaster/TestDelegationMaster_Statechart ==
  state chart
    state chartRegion [parallel]
      state Main
        state synchronization [parallel]
          state Start
          state Stop
            entry: successAvailableSynchronizationDelMaster = true; failureAvailableSynchronizationDelMaster = true
            exit: successAvailableSynchronizationDelMaster = false; failureAvailableSynchronizationDelMaster = false
          state Failure
          state Success
          Stop -> Failure [order 1] : success
          Stop -> chart.chartRegion.Main.synchronization.Success [order 2] : failure
          Start -> Stop : [synchronizeAvailablePort_delegation_master]{send(synchronize, port_delegation_master)}
        state port_delegation_master [parallel]
          state Inactive
            entry: synchronizeAvailableDelegation_Master = true
            exit: synchronizeAvailableDelegation_Master = false
          state Success
          state Fail
          state Running
            entry: reset(c0)
          state Inv_Error
          Running -> chart.chartRegion.Main.port_delegation_master.Success [order 2] : [[checkQueue(EVT_COMPLETED, delegation_masterEvtReadOut)]]
          Running -> Fail [order 1] : [[checkQueue(EVT_FAILED, delegation_masterEvtReadOut)]]
          Inactive -> Running : synchronize{[delegation_masterEvtWriteOut, delegation_masterParamWriteOut] = enqueue(EVT_DELEGATE, delegation_masterEvtWriteOut, delegation_masterParamWriteOut)}
          chart.chartRegion.Main.port_delegation_master.Success -> Inactive : [successAvailableSynchronization]{send(success, synchronization)}
          Fail -> Inactive : [failureAvailableSynchronization]{send(failure, synchronization)}
          Running -> Inv_Error [order 3] : [time(c0) > 10]
    state DataInit [parallel]
    DataInit -> DataInit : {delegation_masterEvtWriteOut = delegation_masterEvtWriteIn;
        | delegation_masterParamWriteOut = delegation_masterParamWriteIn;
        | delegation_masterEvtReadOut = delegation_masterEvtReadIn;
        | delegation_masterParamReadOut = delegation_masterParamReadIn;
        | }
  (default) -> Start
  (default) -> Inactive
  (default) -> Main
  (default) -> chart
  data: EVT_COMPLETED constant uint32 =3; EVT_FAILED constant uint32 =4; EVT_DELEGATE constant uint32 =2; c0 local double =0.0; EVT_DELEGATE constant uint32 =2; EVT_COMPLETED constant uint32 =3; EVT_FAILED constant uint32 =4; successAvailableSynchronizationDelMaster local boolean =false; failureAvailableSynchronizationDelMaster local boolean =false; synchronizeAvailableDelegation_Master local boolean =false; evtQueueIn function_input; param function_input; paramQueueIn function_input; event function_input; evtQueue function_output; paramQueue function_output; event function_input; evtQueue function_input; available function_output; event function_input; evtQueueIn function_input; paramQueueIn function_input; evtQueue function_output; paramQueue function_output; parameter function_output; clock function_input; logicalTime function_output; clock function_input; clockSignal input; delegation_masterReadIn input; delegation_masterParamReadIn input; delegation_masterWriteIn input; delegation_masterParamWriteIn input; delegation_masterReadOut output; delegation_masterParamReadOut output; delegation_masterWriteOut output; delegation_masterParamWriteOut output
  events: synchronize local EITHER_EDGE_EVENT; success local EITHER_EDGE_EVENT; failure local EITHER_EDGE_EVENT
  function enqueue:
    | function [evtQueue, paramQueue] = enqueue(event, evtQueueIn, param, paramQueueIn) %eml 
    |  evtQueue = evtQueueIn; 
    |  paramQueue = paramQueueIn; 
    |  for i = 1:length(evtQueueIn) 
    |  if evtQueueIn(i) == uint8(0) 
    |  evtQueueIn(i) = event; 
    |  paramQueue(i) = param; 
    |  return 
    |  end 
    |  end
  function checkQueue:
    | function available = checkQueue(event, evtQueue) %eml 
    |  available = false; 
    |  for i = 1:length(evtQueue) 
    |      if evtQueue(i) == event 
    |          available = true;    
    |          return 
    |      end 
    |  end
  function dequeue:
    | function [evtQueue, paramQueue, parameter] = dequeue(event, evtQueueIn, paramQueueIn) %eml 
    |  evtQueue = evtQueueIn; 
    |  paramQueue = paramQueueIn; 
    |  parameter = 0; 
    |  for i = 1:length(evtQueue) 
    |  if evtQueue(i) == event 
    |  parameter = paramQueue(i); 
    |  for j = i:length(evtQueue)-1 
    |   evtQueue(j) = evtQueue(j+1); 
    |  paramQueue(j) = paramQueue(j+1); 
    |  end 
    |  evtQueue(length(evtQueue)) = 0; 
    |  paramQueue(length(paramQueue)) = 0; 
    |  return 
    |  end 
    |  end
  function time:
    | function logicalTime = time(clock) 
    |  sample = 0.01;  % the sample time of the system clock 
    |  %convert to pass units of time after last reset 
    |  logicalTime = uint32((clockSignal - clock)/sample);
  function reset:
    | function reset(clock) 
    |  %set clock variable to current time 
    |  clock = clockSignal;

== stateflow chart TestEventListenerSlave/TestEventListenerSlave_Statechart ==
  state chart
    state chartRegion [parallel]
      state Main
        state synch [parallel]
          state s1
            entry: performedAvailableStatechart = true
            exit: performedAvailableStatechart = false
          s1 -> s1 : performed
        state port eventlistener slave [parallel]
          state Receiving
          Receiving -> Receiving : [([performedAvailableSynch]/) && ([checkQueue(EVT_PERFORM, eventListener_slaveEvtReadOut)])]{send(performed, synch)}
    state DataInit [parallel]
    DataInit -> DataInit : {eventListener_slaveEvtWriteOut = eventListener_slaveEvtWriteIn;
        | eventListener_slaveParamWriteOut = eventListener_slaveParamWriteIn;
        | eventListener_slaveEvtReadOut = eventListener_slaveEvtReadIn;
        | eventListener_slaveParamReadOut = eventListener_slaveParamReadIn;
        | }
  (default) -> s1
  (default) -> Receiving
  (default) -> Main
  (default) -> chart
  data: EVT_PERFORM constant uint32 =1; EVT_PERFORM constant uint32 =1; performedAvailableStatechart local boolean =false; evtQueueIn function_input; param function_input; paramQueueIn function_input; event function_input; evtQueue function_output; paramQueue function_output; event function_input; evtQueue function_input; available function_output; event function_input; evtQueueIn function_input; paramQueueIn function_input; evtQueue function_output; paramQueue function_output; parameter function_output; clock function_input; logicalTime function_output; clock function_input; clockSignal input; eventListener_slaveReadIn input; eventListener_slaveParamReadIn input; eventListener_slaveWriteIn input; eventListener_slaveParamWriteIn input; eventListener_slaveReadOut output; eventListener_slaveParamReadOut output; eventListener_slaveWriteOut output; eventListener_slaveParamWriteOut output
  events: performed local EITHER_EDGE_EVENT
  function enqueue:
    | function [evtQueue, paramQueue] = enqueue(event, evtQueueIn, param, paramQueueIn) %eml 
    |  evtQueue = evtQueueIn; 
    |  paramQueue = paramQueueIn; 
    |  for i = 1:length(evtQueueIn) 
    |  if evtQueueIn(i) == uint8(0) 
    |  evtQueueIn(i) = event; 
    |  paramQueue(i) = param; 
    |  return 
    |  end 
    |  end
  function checkQueue:
    | function available = checkQueue(event, evtQueue) %eml 
    |  available = false; 
    |  for i = 1:length(evtQueue) 
    |      if evtQueue(i) == event 
    |          available = true;    
    |          return 
    |      end 
    |  end
  function dequeue:
    | function [evtQueue, paramQueue, parameter] = dequeue(event, evtQueueIn, paramQueueIn) %eml 
    |  evtQueue = evtQueueIn; 
    |  paramQueue = paramQueueIn; 
    |  parameter = 0; 
    |  for i = 1:length(evtQueue) 
    |  if evtQueue(i) == event 
    |  parameter = paramQueue(i); 
    |  for j = i:length(evtQueue)-1 
    |   evtQueue(j) = evtQueue(j+1); 
    |  paramQueue(j) = paramQueue(j+1); 
    |  end 
    |  evtQueue(length(evtQueue)) = 0; 
    |  paramQueue(length(paramQueue)) = 0; 
    |  return 
    |  end 
    |  end
  function time:
    | function logicalTime = time(clock) 
    |  sample = 0.01;  % the sample time of the system clock 
    |  %convert to pass units of time after last reset 
    |  logicalTime = uint32((clockSignal - clock)/sample);
  function reset:
    | function reset(clock) 
    |  %set clock variable to current time 
    |  clock = clockSignal;

== stateflow chart TestEventListenerMaster/TestEventListenerMaster_Statechart ==
  state chart
    state chartRegion [parallel]
      state Main
        state synch [parallel]
          state s1
          state s2
          s1 -> s2 : [performAvailableEventListenerMaster]{send(perform, eventListenerMaster)}
        state eventListenerMaster [parallel]
          state Waiting
            entry: performAvailableEventListener_Master = true
            exit: performAvailableEventListener_Master = false
          Waiting -> Waiting : perform{[eventListener_masterEvtWriteOut, eventListener_masterParamWriteOut] = enqueue(EVT_PERFORM, eventListener_masterEvtWriteOut, eventListener_masterParamWriteOut)}
    state DataInit [parallel]
    DataInit -> DataInit : {eventListener_masterEvtWriteOut = eventListener_masterEvtWriteIn;
        | eventListener_masterParamWriteOut = eventListener_masterParamWriteIn;
        | eventListener_masterEvtReadOut = eventListener_masterEvtReadIn;
        | eventListener_masterParamReadOut = eventListener_masterParamReadIn;
        | }
  (default) -> s1
  (default) -> Waiting
  (default) -> Main
  (default) -> chart
  data: EVT_PERFORM constant uint32 =1; EVT_PERFORM constant uint32 =1; performAvailableEventListener_Master local boolean =false; evtQueueIn function_input; param function_input; paramQueueIn function_input; event function_input; evtQueue function_output; paramQueue function_output; event function_input; evtQueue function_input; available function_output; event function_input; evtQueueIn function_input; paramQueueIn function_input; evtQueue function_output; paramQueue function_output; parameter function_output; clock function_input; logicalTime function_output; clock function_input; clockSignal input; eventListener_masterReadIn input; eventListener_masterParamReadIn input; eventListener_masterWriteIn input; eventListener_masterParamWriteIn input; eventListener_masterReadOut output; eventListener_masterParamReadOut output; eventListener_masterWriteOut output; eventListener_masterParamWriteOut output
  events: perform local EITHER_EDGE_EVENT
  function enqueue:
    | function [evtQueue, paramQueue] = enqueue(event, evtQueueIn, param, paramQueueIn) %eml 
    |  evtQueue = evtQueueIn; 
    |  paramQueue = paramQueueIn; 
    |  for i = 1:length(evtQueueIn) 
    |  if evtQueueIn(i) == uint8(0) 
    |  evtQueueIn(i) = event; 
    |  paramQueue(i) = param; 
    |  return 
    |  end 
    |  end
  function checkQueue:
    | function available = checkQueue(event, evtQueue) %eml 
    |  available = false; 
    |  for i = 1:length(evtQueue) 
    |      if evtQueue(i) == event 
    |          available = true;    
    |          return 
    |      end 
    |  end
  function dequeue:
    | function [evtQueue, paramQueue, parameter] = dequeue(event, evtQueueIn, paramQueueIn) %eml 
    |  evtQueue = evtQueueIn; 
    |  paramQueue = paramQueueIn; 
    |  parameter = 0; 
    |  for i = 1:length(evtQueue) 
    |  if evtQueue(i) == event 
    |  parameter = paramQueue(i); 
    |  for j = i:length(evtQueue)-1 
    |   evtQueue(j) = evtQueue(j+1); 
    |  paramQueue(j) = paramQueue(j+1); 
    |  end 
    |  evtQueue(length(evtQueue)) = 0; 
    |  paramQueue(length(paramQueue)) = 0; 
    |  return 
    |  end 
    |  end
  function time:
    | function logicalTime = time(clock) 
    |  sample = 0.01;  % the sample time of the system clock 
    |  %convert to pass units of time after last reset 
    |  logicalTime = uint32((clockSignal - clock)/sample);
  function reset:
    | function reset(clock) 
    |  %set clock variable to current time 
    |  clock = clockSignal;
